simulink model "Misil_Simulink_bus"  (R2021b)
settings: Solver=VariableStepAuto  StartTime=0.0  StopTime=10  FixedStep=0.001  RelTol=1e-3  EnableMultiTasking=on
PreLoadFcn:
  | codigos
libraries: aerolibanim x1, aerolibatmos2 x1
settings Model: Creator=usuario  LastModifiedBy=verti
settings SolverCC: AlgebraicLoopSolver=TrustRegion
settings DataIOCC: LimitDataPoints=on  SaveFormat=Array  SignalLoggingSaveFormat=ModelDataLogs  ReturnWorkspaceOutputs=off
settings OptimizationCC: ExpressionDepthLimit=2147483647  LifeSpan=inf
settings DebuggingCC: UnderspecifiedInitializationDetection=Classic  MergeDetectMultiDrivingBlocksExec=none  SolverPrmCheckMsg=warning  FcnCallInpInsideContextMsg=warning  StateNameClashWarn=warning  SFUnexpectedBacktrackingDiag=warning  SFNoUnconditionalDefaultTransitionDiag=warning  SFExecutionAtInitializationDiag=none  SFMachineParentedDataDiag=warning  ArithmeticOperatorsInVariantConditions=warning
settings HardwareCC: ProdBitPerPointer=32  ProdBitPerSizeT=32  ProdBitPerPtrDiffT=32  ProdLargestAtomicFloat=None  ProdIntDivRoundTo=Undefined  ProdEndianess=Unspecified  ProdWordSize=32  ProdHWDeviceType=32-bit Generic
settings ModelReferenceCC: PropagateSignalLabelsOutOfModel=off
settings SFSimCC: SimUseLocalCustomCode=off  CustomCodeUndefinedFunction=UseInterfaceOnly
settings RTWCC: RTWUseLocalCustomCode=off
settings CodeAppCC: StateflowObjectComments=on
settings GRTTargetCC: TargetLangStandard=C89/C90 (ANSI)  CombineOutputUpdateFcns=off  GRTInterface=on
settings ConfigComp: CovMetricSettings=dw  CovSaveCumulativeToWorkspaceVar=on  CovSaveSingleToWorkspaceVar=on  CovExternalEMLEnable=off

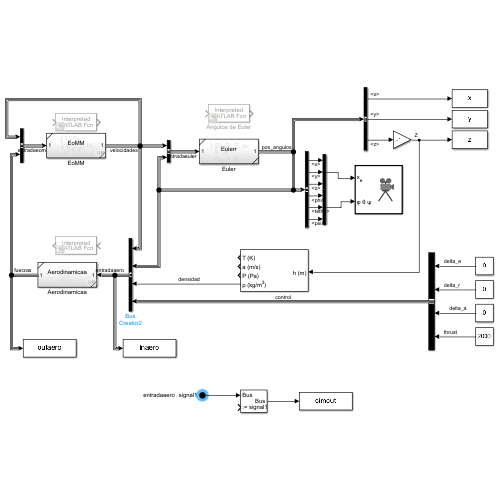
[thumbnail: Simulink's stored preview of the top-level diagram]
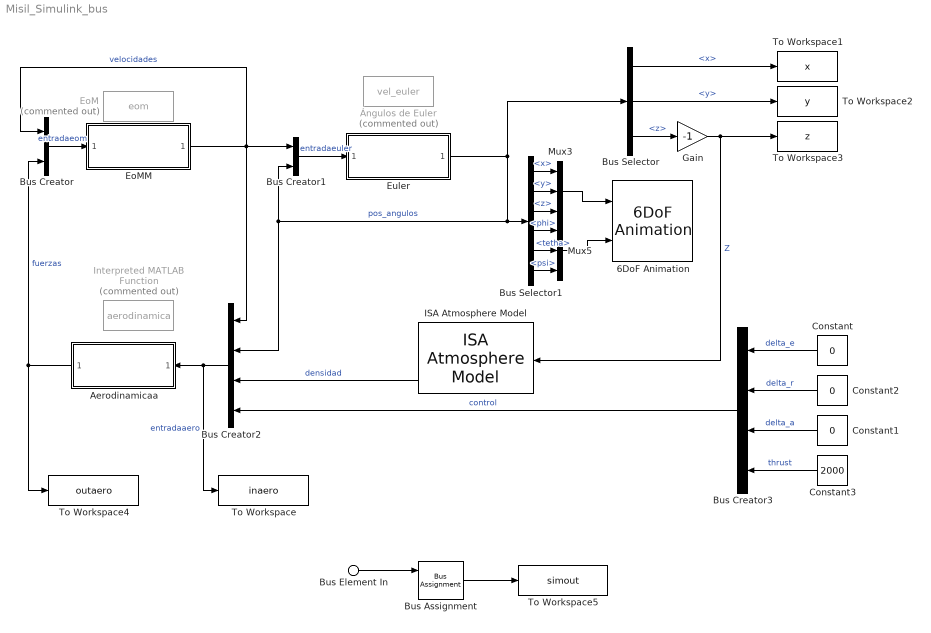
== system Misil_Simulink_bus ==
  Bus Element In : Inport  PortName=entradaaero  Element=signal1
  6DoF Animation : aerolibanim/6DoF Animation  u1=[0 4000 0 4000 0 4000]  u2=0.1  u3=20  u4=[0 0 0]  u5=Fly alongside  u6=[200 200 200]  u7=10  u8=on
  Aerodinamicaa : Subsystem  ReferencedSubsystem=Aerodinamicaa
  Bus Assignment : BusAssignment  AssignedSignals=signal1
  Bus Creator : BusCreator  Inputs=2
  Bus Creator1 : BusCreator  Inputs=2
  Bus Creator2 : BusCreator  Inputs=4
  Bus Creator3 : BusCreator  Inputs=4
  Bus Selector : BusSelector  OutputSignals=x,y,z
  Bus Selector1 : BusSelector  OutputSignals=x,y,z,phi,tetha,psi
  Constant : Constant  Value=0
  Constant1 : Constant  Value=0
  Constant2 : Constant  Value=0
  Constant3 : Constant  Value=2000
  EoM : MATLABFcn  Commented=on  MATLABFcn=eom  OutputDimensions=6
  EoMM : Subsystem  ReferencedSubsystem=EoMM
  Euler : Subsystem  ReferencedSubsystem=Eulerr
  Gain : Gain  Gain=-1
  ISA Atmosphere Model : aerolibatmos2/ISA Atmosphere Model  custom=off  g=9.80665  gamma=1.4  R=287.0531  L=0.0065  h_trop=11000  h_strat=20000  rho0=1.225  P0=101325  T0=288.15  h0=0
  Interpreted MATLAB Function : MATLABFcn  Commented=on  MATLABFcn=aerodinamica  OutputDimensions=6
  Mux3 : Mux  Inputs=3
  Mux5 : Mux  Inputs=3
  To Workspace : ToWorkspace  VariableName=inaero  SaveFormat=Timeseries  SampleTime=-1
  To Workspace1 : ToWorkspace  VariableName=x  SampleTime=-1
  To Workspace2 : ToWorkspace  VariableName=y  SampleTime=-1
  To Workspace3 : ToWorkspace  VariableName=z  SampleTime=-1
  To Workspace4 : ToWorkspace  VariableName=outaero  SaveFormat=Timeseries  SampleTime=-1
  To Workspace5 : ToWorkspace  VariableName=simout  SaveFormat=Timeseries  SampleTime=-1
  Ángulos de Euler : MATLABFcn  Commented=on  MATLABFcn=vel_euler  OutputDimensions=6
  wires:
  EoMM/1 -> Bus Creator2/1, Bus Creator1/1, Bus Creator/1  "velocidades"
  Euler/1 -> Bus Selector/1, Bus Creator1/2, Bus Creator2/2, Bus Selector1/1  "pos_angulos"
  Bus Selector/3 -> Gain/1  "<z>"
  Gain/1 -> To Workspace3/1, ISA Atmosphere Model/1  "Z"
  Bus Selector/1 -> To Workspace1/1  "<x>"
  Bus Selector/2 -> To Workspace2/1  "<y>"
  Constant3/1 -> Bus Creator3/4  "thrust"
  Constant1/1 -> Bus Creator3/3  "delta_a"
  Constant2/1 -> Bus Creator3/2  "delta_r"
  Constant/1 -> Bus Creator3/1  "delta_e"
  ISA Atmosphere Model/4 -> Bus Creator2/3  "densidad"
  Aerodinamicaa/1 -> Bus Creator/2, To Workspace4/1  "fuerzas"
  Bus Selector1/2 -> Mux3/2  "<y>"
  Bus Selector1/3 -> Mux3/3  "<z>"
  Bus Selector1/1 -> Mux3/1  "<x>"
  Mux3/1 -> 6DoF Animation/1
  Bus Selector1/4 -> Mux5/1  "<phi>"
  Bus Selector1/5 -> Mux5/2  "<tetha>"
  Bus Selector1/6 -> Mux5/3  "<psi>"
  Mux5/1 -> 6DoF Animation/2
  Bus Creator/1 -> EoMM/1  "entradaeom"
  Bus Creator1/1 -> Euler/1  "entradaeuler"
  Bus Creator2/1 -> To Workspace/1, Aerodinamicaa/1  "entradaaero"
  Bus Creator3/1 -> Bus Creator2/4  "control"
  Bus Element In/1 -> Bus Assignment/1
  Bus Assignment/1 -> To Workspace5/1
